simulink model "mcb_pmsm_foc_test_f28379d"  (R2023b)
settings: Solver=FixedStepDiscrete  StartTime=0.0  StopTime=10  RelTol=1e-3  EnableMultiTasking=on
InitFcn:
  | mcb_pmsm_foc_test_f28379d_data;
values from neighbouring files (symbols this model uses):
  dataType = 'single'    [mcb_pmsm_foc_sensorless_f28379d_datascript.m]    (also in mcb_pmsm_foc_test_f28379d_data.m)
  inverter = mcb_updateInverterParameters(pmsm,inverter,target)    [mcb_pmsm_foc_sensorless_f28379d_datascript.m]    (also in mcb_pmsm_foc_test_f28379d_data.m)
  PI_params = mcb_SetControllerParameters(pmsm,inverter,PU_System,T_pwm,2*Ts,Ts_speed)    [mcb_pmsm_foc_sensorless_f28379d_datascript.m]    (also in mcb_pmsm_foc_test_f28379d_data.m = mcb_SetControllerParameters(pmsm,inverter,PU_System,T_pwm,Ts)
  pmsm = mcb_SetPMSMMotorParameters("new")    [mcb_pmsm_foc_sensorless_f28379d_datascript.m]    (also in mcb_pmsm_foc_test_f28379d_data.m = mcb_SetPMSMMotorParameters("SF2804"))
  PU_System = mcb_SetPUSystem(pmsm,inverter)    [mcb_pmsm_foc_sensorless_f28379d_datascript.m]    (also in mcb_pmsm_foc_test_f28379d_data.m)
  target = mcb_SetProcessorDetails('F28379D',PWM_frequency)    [mcb_pmsm_foc_sensorless_f28379d_datascript.m]    (also in mcb_pmsm_foc_test_f28379d_data.m)
  Ts = T_pwm    [discrete_tansfer_fcn.m]    (also in mcb_pmsm_foc_sensorless_f28379d_datascript.m = 5e-05; mcb_pmsm_foc_test_f28379d_data.m = 5e-05)
  Ts_motor = T_pwm/2    (= 2.5e-05)    [mcb_pmsm_foc_sensorless_f28379d_datascript.m]    (also in mcb_pmsm_foc_test_f28379d_data.m)
  Ts_sensor = 20*Ts    (= 0.001)    [mcb_pmsm_foc_sensorless_f28379d_datascript.m]    (also in mcb_pmsm_foc_test_f28379d_data.m; virtual_speed.m)
  Ts_simulink = T_pwm/2    (= 2.5e-05)    [mcb_pmsm_foc_sensorless_f28379d_datascript.m]    (also in mcb_pmsm_foc_test_f28379d_data.m)
  Ts_speed = 20*Ts    (= 0.001)    [mcb_pmsm_foc_sensorless_f28379d_datascript.m]    (also in mcb_pmsm_foc_test_f28379d_data.m = 0.0005)
undefined symbols (not defined in the file or in its folder): DiscIntNeverNeededParam, Down, GPTRIP1SEL, GPTRIP2SEL, TZ1, TZ2, Up
libraries: c280xlib x14, simulink x11, mcbcontrolslib x9, c2802xlib x7, slpidlib x5, c2837xDlib x4, mcbpositiondecoderlib x3, canmsglib x2, svdschedulerlib x2, dspsigops x1, svdutilitieslib x1, mcbplantlib x1
(part 3 of 3)

== system mcb_pmsm_foc_test_f28379d/Serial Receive/SCI_Rx/Simulation ==
  Data Type Conversion2 : DataTypeConversion  OutDataTypeStr=dataType  RndMeth=Simplest  SaturateOnIntegerOverflow=off
  Data_Conditioning_Tx : Subsystem  Variant=on
  Debug_signals : Constant  OutDataTypeStr=uint16  SampleTime=-1
  Enable : Constant  OutDataTypeStr=uint16  SampleTime=-1
  Parse : Subsystem
  Reversal : Step  Time=3
  Speed_Ref_Final (rpm) : Constant  Value=-0.8*pmsm.N_base  OutDataTypeStr=dataType  SampleTime=-1
  Speed_Ref_Init (rpm) : Step  Before=0.2*pmsm.N_base  After=0.9*pmsm.N_base
  Switch : Switch  Criteria=u2 > Threshold  SaturateOnIntegerOverflow=off  InputSameDT=off
  rpm2PU : Gain  Gain=1/pmsm.N_base  RndMeth=Simplest  OutDataTypeStr=Inherit: Same as input
  Data : Outport
  wires:
  Data_Conditioning_Tx/1(Data) -> Data/1
  Parse/1(Data) -> Data_Conditioning_Tx/2(In2)
  Data Type Conversion2/1 -> Data_Conditioning_Tx/1(In1)
  Enable/1 -> Parse/1(Enable_PWM)
  Debug_signals/1 -> Parse/2(Debug_signals)
  rpm2PU/1 -> Data Type Conversion2/1
  Switch/1 -> rpm2PU/1
  Speed_Ref_Final (rpm)/1 -> Switch/1
  Reversal/1 -> Switch/2
  Speed_Ref_Init (rpm)/1 -> Switch/3

== system mcb_pmsm_foc_test_f28379d/Speed Control/PI_Controller_Speed1/Switch Case Action Subsystem ==
  Action Port : ActionPort  ActionPortLabel=case [ 1 ]:
  Constant : Constant  Value=0  OutDataTypeStr=single
  Constant1 : Constant  Value=0  OutDataTypeStr=single
  Constant2 : Constant  Value=0  OutDataTypeStr=boolean
  theta_virtual : Outport
  Iq_ref* : Outport  Port=2
  CloseLoop_Enable : Outport  Port=3
  wires:
  Constant/1 -> theta_virtual/1
  Constant1/1 -> Iq_ref*/1
  Constant2/1 -> CloseLoop_Enable/1

== system mcb_pmsm_foc_test_f28379d/Speed Control/PI_Controller_Speed1/Switch Case Action Subsystem1 ==
  Iq_ref : Inport
  Action Port : ActionPort  ActionPortLabel=case [ 2 ]:
  Constant : Constant  Value=0  OutDataTypeStr=single
  Constant2 : Constant  Value=0  OutDataTypeStr=boolean
  theta_virtual : Outport
  Iq_ref* : Outport  Port=2
  CloseLoop_Enable : Outport  Port=3
  wires:
  Constant/1 -> theta_virtual/1
  Iq_ref/1 -> Iq_ref*/1
  Constant2/1 -> CloseLoop_Enable/1

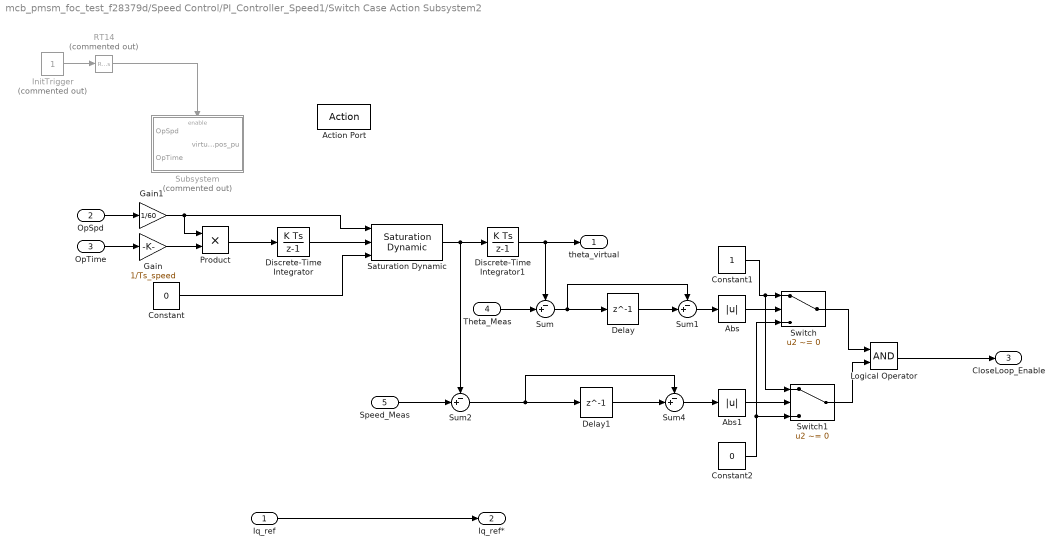
== system mcb_pmsm_foc_test_f28379d/Speed Control/PI_Controller_Speed1/Switch Case Action Subsystem2 ==
  Iq_ref : Inport
  OpSpd : Inport  Port=2
  OpTime : Inport  Port=3
  Theta_Meas : Inport  Port=4
  Speed_Meas : Inport  Port=5
  Action Port : ActionPort  ActionPortLabel=case [ 3 ]:
  Abs : Abs  SaturateOnIntegerOverflow=off
  Abs1 : Abs  SaturateOnIntegerOverflow=off
  Constant : Constant  Value=0
  Constant1 : Constant  OutDataTypeStr=boolean
  Constant2 : Constant  Value=0  OutDataTypeStr=boolean
  Delay : Delay  DelayLength=1  InitialCondition=0
  Delay1 : Delay  DelayLength=1  InitialCondition=0
  Discrete-Time Integrator : DiscreteIntegrator  SampleTime=-1  OutDataTypeStr=single  ICPrevOutput=DiscIntNeverNeededParam  ICPrevScaledInput=DiscIntNeverNeededParam
  Discrete-Time Integrator1 : DiscreteIntegrator  SampleTime=-1  OutDataTypeStr=single  ICPrevOutput=DiscIntNeverNeededParam  ICPrevScaledInput=DiscIntNeverNeededParam
  Gain : Gain  Gain=1/Ts_speed
  Gain1 : Gain  Gain=1/60
  InitTrigger : Constant  Priority=10  Commented=on  OutDataTypeStr=boolean
  Logical Operator : Logic  AllPortsSameDT=off  OutDataTypeStr=boolean
  Product : Product  OutDataTypeStr=single
  RT14 : RateTransition  Commented=on  Deterministic=off  OutPortSampleTime=Ts_sensor
  Saturation Dynamic : simulink/Discontinuities/Saturation Dynamic  OutMin=[]  OutMax=[]  OutDataTypeStr=single  OutDataType=fixdt(1, 16)  OutScaling=2^-10  DoSatur=off
  Subsystem : Subsystem  Commented=on
  Sum{,1..2,4} (4 alike) : Sum  Inputs=-+|
  Switch : Switch  Criteria=u2 ~= 0  SaturateOnIntegerOverflow=off  InputSameDT=off
  Switch1 : Switch  Criteria=u2 ~= 0  SaturateOnIntegerOverflow=off  InputSameDT=off
  theta_virtual : Outport
  Iq_ref* : Outport  Port=2
  CloseLoop_Enable : Outport  Port=3
  wires:
  Iq_ref/1 -> Iq_ref*/1
  InitTrigger/1 -> RT14/1
  RT14/1 -> Subsystem/Enable
  Constant/1 -> Saturation Dynamic/3
  OpSpd/1 -> Gain1/1
  Gain/1 -> Product/2
  OpTime/1 -> Gain/1
  Product/1 -> Discrete-Time Integrator/1
  Gain1/1 -> Saturation Dynamic/1, Product/1
  Discrete-Time Integrator/1 -> Saturation Dynamic/2
  Saturation Dynamic/1 -> Sum2/1, Discrete-Time Integrator1/1
  Discrete-Time Integrator1/1 -> Sum/1, theta_virtual/1
  Theta_Meas/1 -> Sum/2
  Speed_Meas/1 -> Sum2/2
  Sum/1 -> Sum1/1, Delay/1
  Delay/1 -> Sum1/2
  Sum1/1 -> Abs/1
  Abs/1 -> Switch/2
  Switch/1 -> Logical Operator/1
  Logical Operator/1 -> CloseLoop_Enable/1
  Switch1/1 -> Logical Operator/2
  Constant1/1 -> Switch1/1, Switch/1
  Abs1/1 -> Switch1/2
  Delay1/1 -> Sum4/2
  Constant2/1 -> Switch/3, Switch1/3
  Sum4/1 -> Abs1/1
  Sum2/1 -> Sum4/1, Delay1/1

== system mcb_pmsm_foc_test_f28379d/Speed Control/PI_Controller_Speed1/Switch Case Action Subsystem3 ==
  Iq_ref : Inport
  Action Port : ActionPort  ActionPortLabel=case [ 4 ]:
  Constant2 : Constant  Value=0  OutDataTypeStr=boolean
  theta_virtual : Outport
  Iq_ref* : Outport  Port=2
  CloseLoop_Enable : Outport  Port=3
  wires:
  ? -> theta_virtual/1
  Iq_ref/1 -> Iq_ref*/1
  Constant2/1 -> CloseLoop_Enable/1

== system mcb_pmsm_foc_test_f28379d/Speed Control/POS_Loop/Subsystem ==
  In1 : Inport
  Action Port : ActionPort  ActionPortLabel=if(u1 > 0.5)
  Fcn : Fcn  Expr=u(1)-1
  Out1 : Outport
  wires:
  In1/1 -> Fcn/1
  Fcn/1 -> Out1/1

== system mcb_pmsm_foc_test_f28379d/Speed Control/POS_Loop/Subsystem1 ==
  In1 : Inport
  Action Port : ActionPort  ActionPortLabel=elseif(u1 < -0.5)
  Fcn1 : Fcn  Expr=u(1)+1
  Out1 : Outport
  wires:
  Fcn1/1 -> Out1/1
  In1/1 -> Fcn1/1

== system mcb_pmsm_foc_test_f28379d/Speed Control/POS_Loop/Subsystem2 ==
  In1 : Inport
  Action Port : ActionPort  ActionPortLabel=else
  Out1 : Outport
  wires:
  In1/1 -> Out1/1

== system mcb_pmsm_foc_test_f28379d/AS5600 Read/Initialization/Delay 1ms/System Outputs ==

== system mcb_pmsm_foc_test_f28379d/Current Control/Control_System/Current_Controllers/PI_Controller_Id ==
  I_ref : Inport
  I_fb : Inport  Port=2
  Data Store Read1 : DataStoreRead  DataStoreName=Enable  IndexOptions=Index vector (dialog)  Indices=1  OutputSizes=1
  Discrete PI Controller with anti-windup & reset : slpidlib/PID Controller  Controller=PI  Form=Parallel  TimeDomain=Discrete-time  UseExternalTs=off  SampleTime=-1  IntegratorMethod=Forward Euler  FilterMethod=Forward Euler  ControllerParametersSource=external  P=1  I=1  UseKiTs=on  D=0  N=100  UseFilter=on  TunerSelectOption=Transfer Function Based (PID Tuner App)  InitialConditionSource=external  InitialConditionForIntegrator=0  InitialConditionForFilter=0  DifferentiatorICPrevScaledInput=0  ExternalReset=level  TrackingMode=off  Kt=1  LimitOutput=on  SatLimitsSource=internal  UpperSaturationLimit=1  LowerSaturationLimit=-1  LinearizeAsGain=on  AntiWindupMode=clamping  Kb=1  LimitIntegrator=off  UpperIntegratorSaturationLimit=inf  LowerIntegratorSaturationLimit=-inf  RndMeth=Simplest  POutMin=[]  POutMax=[]  IOutMin=[]  IOutMax=[]  DOutMin=[]  DOutMax=[]  NOutMin=[]  NOutMax=[]  SumOutMin=[]  SumOutMax=[]  SaturationOutDataTypeStr=Inherit: Inherit via back propagation  SaturationOutMin=[]  SaturationOutMax=[]  PParamMin=[]  PParamMax=[]  IParamMin=[]  IParamMax=[]  DParamMin=[]  DParamMax=[]  NParamMin=[]  NParamMax=[]  KbParamMin=[]  KbParamMax=[]  KtParamMin=[]  KtParamMax=[]  KbOutMin=[]  KbOutMax=[]  KtOutMin=[]  KtOutMax=[]  IntegratorOutMin=[]  IntegratorOutMax=[]  FilterOutMin=[]  FilterOutMax=[]  SumI1OutMin=[]  SumI1OutMax=[]  SumI2OutMin=[]  SumI2OutMax=[]  SumI3OutMin=[]  SumI3OutMax=[]  SumI4OutMin=[]  SumI4OutMax=[]  SumDOutMin=[]  SumDOutMax=[]  DifferentiatorOutMin=[]  DifferentiatorOutMax=[]  FilterDiffOutCoefMin=[]  FilterDiffOutCoefMax=[]  ReciprocalOutMin=[]  ReciprocalOutMax=[]  SumDenOutMin=[]  SumDenOutMax=[]  SumNumOutMin=[]  SumNumOutMax=[]  DivideOutMin=[]  DivideOutMax=[]  UdiffTsProdOutMin=[]  UdiffTsProdOutMax=[]  NTsProdOutMin=[]  NTsProdOutMax=[]  UintegralTsProdOutMin=[]  UintegralTsProdOutMax=[]  UngainTsProdOutMin=[]  UngainTsProdOutMax=[]  ClampingZeroOutDataTypeStr=Inherit: Inherit via back propagation  ClampingZeroOutMin=[]  ClampingZeroOutMax=[]  FilterDenConstantOutDataTypeStr=Inherit: Inherit via back propagation  FilterDenConstantOutMin=[]  FilterDenConstantOutMax=[]  PCopyOutDataTypeStr=Inherit: Inherit via back propagation  PCopyOutMin=[]  PCopyOutMax=[]  NCopyOutDataTypeStr=Inherit: Inherit via back propagation  NCopyOutMin=[]  NCopyOutMax=[]  IntegratorContinuousStateAttributes=''  IntegratorStateMustResolveToSignalObject=off  IntegratorRTWStateStorageClass=Auto  FilterContinuousStateAttributes=''  FilterStateMustResolveToSignalObject=off  FilterRTWStateStorageClass=Auto  ParallelPVariant=ExternalParameters  IdealPVariant=Disabled  IVariant=ExternalParameters  DVariant=Disabled  IntegratorVariant=Discrete  SatVariant=Enabled  AWVariant=DiscClampingParallel  PCopyVariant=Disabled  TRVariant=Disabled  FdbkBlocksVariant=Forward  IdealPFdbkVariant=Disabled  SatFdbkVariant=Disabled  DerivativeFilterVariant=Disabled  NVariant=Disabled  NCopyVariant=Disabled_SignalSpec  FilterICVariant=Disabled  IntegratorICVariant=ExternalICs  ExternalResetVariant=ExternalReset  TRSumVariant=Passthrough  SumFdbkVariant=Disabled  SumVariant=Sum_PI  TsampFilterVariant=InternalTs  TsampNgainVariant=Passthrough  TsampIntegralVariant=Disabled_SignalSpec  ExternalSaturationOutDataTypeStr=Inherit: Same as second input
      settings: LibrarySourceBlock=mcbcontrolslib/PI Controller
  Ki : Constant  Value=PI_params.Ki_id*Ts  OutDataTypeStr=dataType  SampleTime=-1
  Ki1 : Constant  Value=0  OutDataTypeStr=dataType  SampleTime=-1
  Kp : Constant  Value=PI_params.Kp_id  OutDataTypeStr=dataType  SampleTime=-1
  Logical Operator : Logic  Operator=NOT  IconShape=distinctive  AllPortsSameDT=off  OutDataTypeStr=boolean
  Sum : Sum  Inputs=|+-  OutDataTypeStr=Inherit: Same as first input
  V_ref : Outport  VectorParamsAs1DForOutWhenUnconnected=off
  wires:
  I_ref/1 -> Sum/1
  I_fb/1 -> Sum/2
  Data Store Read1/1 -> Logical Operator/1
  Discrete PI Controller with anti-windup & reset/1 -> V_ref/1
  Sum/1 -> Discrete PI Controller with anti-windup & reset/1
  Kp/1 -> Discrete PI Controller with anti-windup & reset/2
  Ki/1 -> Discrete PI Controller with anti-windup & reset/3
  Logical Operator/1 -> Discrete PI Controller with anti-windup & reset/4
  Ki1/1 -> Discrete PI Controller with anti-windup & reset/5

== system mcb_pmsm_foc_test_f28379d/Current Control/Control_System/Current_Controllers/PI_Controller_Iq ==
  I_ref : Inport
  I_fb : Inport  Port=2
  Data Store Read1 : DataStoreRead  DataStoreName=Enable  IndexOptions=Index vector (dialog)  Indices=1  OutputSizes=1
  Discrete PI Controller with anti-windup & reset : slpidlib/PID Controller  Controller=PI  Form=Parallel  TimeDomain=Discrete-time  UseExternalTs=off  SampleTime=-1  IntegratorMethod=Forward Euler  FilterMethod=Forward Euler  ControllerParametersSource=external  P=1  I=1  UseKiTs=on  D=0  N=100  UseFilter=on  TunerSelectOption=Transfer Function Based (PID Tuner App)  InitialConditionSource=external  InitialConditionForIntegrator=0  InitialConditionForFilter=0  DifferentiatorICPrevScaledInput=0  ExternalReset=level  TrackingMode=off  Kt=1  LimitOutput=on  SatLimitsSource=internal  UpperSaturationLimit=1  LowerSaturationLimit=-1  LinearizeAsGain=on  AntiWindupMode=clamping  Kb=1  LimitIntegrator=off  UpperIntegratorSaturationLimit=inf  LowerIntegratorSaturationLimit=-inf  RndMeth=Simplest  POutMin=[]  POutMax=[]  IOutMin=[]  IOutMax=[]  DOutMin=[]  DOutMax=[]  NOutMin=[]  NOutMax=[]  SumOutMin=[]  SumOutMax=[]  SaturationOutDataTypeStr=Inherit: Inherit via back propagation  SaturationOutMin=[]  SaturationOutMax=[]  PParamMin=[]  PParamMax=[]  IParamMin=[]  IParamMax=[]  DParamMin=[]  DParamMax=[]  NParamMin=[]  NParamMax=[]  KbParamMin=[]  KbParamMax=[]  KtParamMin=[]  KtParamMax=[]  KbOutMin=[]  KbOutMax=[]  KtOutMin=[]  KtOutMax=[]  IntegratorOutMin=[]  IntegratorOutMax=[]  FilterOutMin=[]  FilterOutMax=[]  SumI1OutMin=[]  SumI1OutMax=[]  SumI2OutMin=[]  SumI2OutMax=[]  SumI3OutMin=[]  SumI3OutMax=[]  SumI4OutMin=[]  SumI4OutMax=[]  SumDOutMin=[]  SumDOutMax=[]  DifferentiatorOutMin=[]  DifferentiatorOutMax=[]  FilterDiffOutCoefMin=[]  FilterDiffOutCoefMax=[]  ReciprocalOutMin=[]  ReciprocalOutMax=[]  SumDenOutMin=[]  SumDenOutMax=[]  SumNumOutMin=[]  SumNumOutMax=[]  DivideOutMin=[]  DivideOutMax=[]  UdiffTsProdOutMin=[]  UdiffTsProdOutMax=[]  NTsProdOutMin=[]  NTsProdOutMax=[]  UintegralTsProdOutMin=[]  UintegralTsProdOutMax=[]  UngainTsProdOutMin=[]  UngainTsProdOutMax=[]  ClampingZeroOutDataTypeStr=Inherit: Inherit via back propagation  ClampingZeroOutMin=[]  ClampingZeroOutMax=[]  FilterDenConstantOutDataTypeStr=Inherit: Inherit via back propagation  FilterDenConstantOutMin=[]  FilterDenConstantOutMax=[]  PCopyOutDataTypeStr=Inherit: Inherit via back propagation  PCopyOutMin=[]  PCopyOutMax=[]  NCopyOutDataTypeStr=Inherit: Inherit via back propagation  NCopyOutMin=[]  NCopyOutMax=[]  IntegratorContinuousStateAttributes=''  IntegratorStateMustResolveToSignalObject=off  IntegratorRTWStateStorageClass=Auto  FilterContinuousStateAttributes=''  FilterStateMustResolveToSignalObject=off  FilterRTWStateStorageClass=Auto  ParallelPVariant=ExternalParameters  IdealPVariant=Disabled  IVariant=ExternalParameters  DVariant=Disabled  IntegratorVariant=Discrete  SatVariant=Enabled  AWVariant=DiscClampingParallel  PCopyVariant=Disabled  TRVariant=Disabled  FdbkBlocksVariant=Forward  IdealPFdbkVariant=Disabled  SatFdbkVariant=Disabled  DerivativeFilterVariant=Disabled  NVariant=Disabled  NCopyVariant=Disabled_SignalSpec  FilterICVariant=Disabled  IntegratorICVariant=ExternalICs  ExternalResetVariant=ExternalReset  TRSumVariant=Passthrough  SumFdbkVariant=Disabled  SumVariant=Sum_PI  TsampFilterVariant=InternalTs  TsampNgainVariant=Passthrough  TsampIntegralVariant=Disabled_SignalSpec  ExternalSaturationOutDataTypeStr=Inherit: Same as second input
      settings: LibrarySourceBlock=mcbcontrolslib/PI Controller
  Ki : Constant  Value=PI_params.Ki_i*Ts  OutDataTypeStr=dataType  SampleTime=-1
  Kp : Constant  Value=PI_params.Kp_i  OutDataTypeStr=dataType  SampleTime=-1
  Kp1 : Constant  Value=0  OutDataTypeStr=dataType  SampleTime=-1
  Logical Operator : Logic  Operator=NOT  IconShape=distinctive  AllPortsSameDT=off  OutDataTypeStr=boolean
  Sum : Sum  Inputs=|+-  OutDataTypeStr=Inherit: Same as first input
  V_ref : Outport  VectorParamsAs1DForOutWhenUnconnected=off
  wires:
  Discrete PI Controller with anti-windup & reset/1 -> V_ref/1
  Data Store Read1/1 -> Logical Operator/1
  I_fb/1 -> Sum/2
  I_ref/1 -> Sum/1
  Kp/1 -> Discrete PI Controller with anti-windup & reset/2
  Sum/1 -> Discrete PI Controller with anti-windup & reset/1
  Ki/1 -> Discrete PI Controller with anti-windup & reset/3
  Logical Operator/1 -> Discrete PI Controller with anti-windup & reset/4
  Kp1/1 -> Discrete PI Controller with anti-windup & reset/5

== system mcb_pmsm_foc_test_f28379d/Current Control/Input Scaling/ Calculate Position and Speed/Subsystem ==
  In1 : Inport
  Action Port : ActionPort  ActionPortLabel=if(u1 > 0.5)
  Fcn : Fcn  Expr=u(1)-1
  Out1 : Outport
  wires:
  In1/1 -> Fcn/1
  Fcn/1 -> Out1/1

== system mcb_pmsm_foc_test_f28379d/Current Control/Input Scaling/ Calculate Position and Speed/Subsystem1 ==
  In1 : Inport
  Action Port : ActionPort  ActionPortLabel=elseif(u1 < -0.5)
  Fcn1 : Fcn  Expr=u(1)+1
  Out1 : Outport
  wires:
  Fcn1/1 -> Out1/1
  In1/1 -> Fcn1/1

== system mcb_pmsm_foc_test_f28379d/Current Control/Input Scaling/ Calculate Position and Speed/Subsystem2 ==
  In1 : Inport
  Action Port : ActionPort  ActionPortLabel=else
  Out1 : Outport
  wires:
  In1/1 -> Out1/1

== system mcb_pmsm_foc_test_f28379d/Current Control/Input Scaling/Calculate Phase Currents/Data_Type ==
  In1 : Inport
  Data_Type_Fixed_Point : Subsystem  VariantControl=~isequal(dataType,'single')
  Data_Type_Float : Subsystem  VariantControl=isequal(dataType,'single')
  Iab_meas_PU : Outport

== system mcb_pmsm_foc_test_f28379d/Current Control/SCI_Tx/Code Generation/Data_Conditioning_Tx ==
  In1 : Inport
  Data_Type_Fixed_Point : Subsystem  VariantControl=~isequal(dataType,'single')
  Data_Type_Float : Subsystem  VariantControl=isequal(dataType, 'single')
  Data_Log : Outport

== system mcb_pmsm_foc_test_f28379d/Current Control/SCI_Tx/Code Generation/Data_Logging ==
  note: Fast Serial Data Monitoring (32-bit)
  Data_Log : Inport
  Counter Limited : simulink/Sources/Counter Limited  uplimit=600-1  tsamp=-1
  Data : Subsystem  TreatAsAtomicUnit=on
  End : Subsystem  TreatAsAtomicUnit=on
  If : If  IfExpression=u1 == 0  ElseIfExpressions=u1 == 599
  Merge : Merge  Inputs=3
  Merge1 : Merge  Inputs=3
  Mux : Mux  Inputs=2
  Start : Subsystem  TreatAsAtomicUnit=on
  Width : Width  OutDataTypeMode=All ports same datatype  DataType=uint16
  SCI_Tx : Outport
  wires:
  If/3 -> Data/Action
  Data/1(Data_out) -> Merge/3
  Width/1 -> Data/2(Data_width), Start/2(Data_width), End/2(Data_width)
  Merge/1 -> Mux/1  "SCI_Tx_Data"
  Counter Limited/1 -> If/1
  Start/2(Iteration) -> Merge1/1
  Start/1(Data_out) -> Merge/1
  If/2 -> End/Action
  Merge1/1 -> Mux/2  "SCI_Tx_Iteration"
  If/1 -> Start/Action
  End/1(Data_out) -> Merge/2
  End/2(Iteration) -> Merge1/2
  Data/2(Iteration) -> Merge1/3
  Mux/1 -> SCI_Tx/1
  Data_Log/1 -> Width/1, Start/1(Data), End/1(Data), Data/1(Data)

== system mcb_pmsm_foc_test_f28379d/Current Control/SCI_Tx/Code Generation/While Iterator Subsystem ==
  Data : Inport
  Iteration : Inport  Port=2
  Add : Sum  Inputs=+-  OutDataTypeStr=Inherit: Same as first input
  Index Vector : MultiPortSwitch  Inputs=1  SaturateOnIntegerOverflow=off  InputSameDT=off
  SCI Transmit : c280xlib/SCI Transmit  sciModule=A  dataHead=''  dataTail=''  frameSize=1  blockingMode=on  outputStatus=off
  While Iterator : WhileIterator  MaxIters=-1  WhileBlockType=do-while  ShowIterationPort=on  OutputDataType=int16
  wires:
  While Iterator/1 -> Add/2, Index Vector/1
  Data/1 -> Index Vector/2
  Index Vector/1 -> SCI Transmit/1
  Add/1 -> While Iterator/1
  Iteration/1 -> Add/1

== system mcb_pmsm_foc_test_f28379d/Hardware Init/Variant Subsystem/Code Generation/Calculate ADC Offset  ==
  Enable : EnablePort
  Constant : Constant  Value=8
  Constant1 : Constant  Value=inverter.CtSensOffsetMax  OutDataTypeStr=Inherit: Inherit via back propagation
  Constant2 : Constant  Value=inverter.CtSensOffsetMin  OutDataTypeStr=Inherit: Inherit via back propagation
  Divide : Product  Inputs=*/  OutDataTypeStr=uint16
  Divide1 : Product  Inputs=*/  OutDataTypeStr=uint16
  For Iterator Subsystem : Subsystem  TreatAsAtomicUnit=on
  If : If  NumInputs=3  IfExpression=u1 > u3 & u1 < u2
  If Action Subsystem : Subsystem  TreatAsAtomicUnit=on
  If Action Subsystem1 : Subsystem  TreatAsAtomicUnit=on
  If Action Subsystem2 : Subsystem  TreatAsAtomicUnit=on
  If Action Subsystem3 : Subsystem  TreatAsAtomicUnit=on
  If1 : If  NumInputs=3  IfExpression=u1 > u3 & u1 < u2
  wires:
  If1/2 -> If Action Subsystem3/Action
  If1/1 -> If Action Subsystem2/Action
  Constant1/1 -> If1/2, If/2
  If/2 -> If Action Subsystem1/Action
  For Iterator Subsystem/1(Out1) -> Divide/1
  If/1 -> If Action Subsystem/Action
  Constant2/1 -> If1/3, If/3
  For Iterator Subsystem/2(Out2) -> Divide1/1
  Divide1/1 -> If1/1, If Action Subsystem2/1(In1)
  Constant/1 -> Divide1/2, Divide/2
  Divide/1 -> If Action Subsystem/1(In1), If/1

== system mcb_pmsm_foc_test_f28379d/Hardware Init/Variant Subsystem/Code Generation/DRV Enable ==
  note: Enable inverter
  In : Inport
  ADC Gain setting : Subsystem
  Constant : Constant  Value=inverter.EnableLogic
  Digital Output : c2837xDlib/Digital Output  Priority=10  GPIO_Number=GPIO120~GPIO127  GPIO_Bit0=off  GPIO_BIT0_Toggle=off  GPIO_Bit1=off  GPIO_BIT1_Toggle=off  GPIO_Bit2=off  GPIO_BIT2_Toggle=off  GPIO_Bit3=off  GPIO_BIT3_Toggle=off  GPIO_Bit4=on  GPIO_BIT4_Toggle=off  GPIO_Bit5=off  GPIO_BIT5_Toggle=off  GPIO_Bit6=off  GPIO_BIT6_Toggle=off  GPIO_Bit7=off  GPIO_BIT7_Toggle=off
  Digital Output1 : c2837xDlib/Digital Output  Priority=10  GPIO_Number=GPIO16~GPIO23  GPIO_Bit0=off  GPIO_BIT0_Toggle=off  GPIO_Bit1=off  GPIO_BIT1_Toggle=off  GPIO_Bit2=off  GPIO_BIT2_Toggle=off  GPIO_Bit3=off  GPIO_BIT3_Toggle=off  GPIO_Bit4=off  GPIO_BIT4_Toggle=off  GPIO_Bit5=off  GPIO_BIT5_Toggle=off  GPIO_Bit6=on  GPIO_BIT6_Toggle=off  GPIO_Bit7=off  GPIO_BIT7_Toggle=off
  Inverter Enable : Constant  OutDataTypeStr=uint16  SampleTime=-1
  NOT : Logic  Operator=NOT  IconShape=distinctive  AllPortsSameDT=off  OutDataTypeStr=boolean
  RunTimeMeasurement : Constant  OutDataTypeStr=uint16  SampleTime=-1
  Switch : Switch  Criteria=u2 > Threshold  SaturateOnIntegerOverflow=off  InputSameDT=off
  wires:
  Inverter Enable/1 -> Switch/1, NOT/1  "Active high logic for inverter enable"
  RunTimeMeasurement/1 -> Digital Output1/1
  Constant/1 -> ADC Gain setting/Enable, Switch/2
  Switch/1 -> Digital Output/1
  NOT/1 -> Switch/3  "Active low logic for inverter enable"
  In/1 -> ADC Gain setting/1(In1)

== system mcb_pmsm_foc_test_f28379d/Hardware Init/Variant Subsystem/Code Generation/Default ADC Offset ==
  Enable : EnablePort
  Constant : Constant  Value=inverter.CtSensAOffset  OutDataTypeStr=Inherit: Inherit via back propagation
  Constant1 : Constant  Value=inverter.CtSensBOffset  OutDataTypeStr=Inherit: Inherit via back propagation
  Data Store Write1 : DataStoreWrite  DataStoreName=IaOffset  IndexOptions=Index vector (dialog)  Indices=1  OutputSizes=1
  Data Store Write2 : DataStoreWrite  DataStoreName=IbOffset  IndexOptions=Index vector (dialog)  Indices=1  OutputSizes=1
  wires:
  Constant/1 -> Data Store Write1/1
  Constant1/1 -> Data Store Write2/1

== system mcb_pmsm_foc_test_f28379d/Serial Receive/SCI_Rx/Code Generation/Data_Type_Fixed_Point ==
  SCI Receive : c280xlib/SCI Receive  sciModule=A  dataHead=''  headerCheckMaxCount=16  dataTail=''  dataType=uint32  dataLenOptions=Length via dialog  dataDim=2  maxDataLength=1  initValue=0  errOption=Output the last received value  errValue=0  sampleTime=-1  blockingMode=on  timeOut=0.00875  outputStatus=off
  Data : Outport
  wires:
  SCI Receive/1 -> Data/1

== system mcb_pmsm_foc_test_f28379d/Serial Receive/SCI_Rx/Code Generation/Data_Type_Float ==
  SCI Receive : c280xlib/SCI Receive  sciModule=A  dataHead=''  headerCheckMaxCount=16  dataTail=''  dataType=single  dataLenOptions=Length via dialog  dataDim=2  maxDataLength=1  initValue=0  errOption=Output the last received value  errValue=0  sampleTime=-1  blockingMode=on  timeOut=0.00875  outputStatus=off
  Data : Outport
  wires:
  SCI Receive/1 -> Data/1

== system mcb_pmsm_foc_test_f28379d/Serial Receive/SCI_Rx/Simulation/Data_Conditioning_Tx ==
  In1 : Inport
  In2 : Inport  Port=2
  Data_Type_Fixed_Point : Subsystem  VariantControl=~isequal(dataType, 'single')
  Data_Type_Float : Subsystem  VariantControl=isequal(dataType, 'single')
  Data : Outport

== system mcb_pmsm_foc_test_f28379d/Serial Receive/SCI_Rx/Simulation/Parse ==
  Enable_PWM : Inport
  Debug_signals : Inport  Port=2
  Bitwise Operator : simulink/Logic and Bit Operations/Bitwise Operator  logicop=AND  UseBitMask=on  BitMask=hex2dec('0001')  BitMaskRealWorld=Stored Integer
  Bitwise Operator1 : simulink/Logic and Bit Operations/Bitwise Operator  logicop=AND  UseBitMask=on  BitMask=hex2dec('00F0')  BitMaskRealWorld=Stored Integer
  Shift Arithmetic1 : ArithShift  BitShiftNumber=-4
  Sum : Sum
  Data : Outport
  wires:
  Bitwise Operator/1 -> Sum/1
  Debug_signals/1 -> Shift Arithmetic1/1
  Sum/1 -> Data/1
  Shift Arithmetic1/1 -> Bitwise Operator1/1
  Enable_PWM/1 -> Bitwise Operator/1
  Bitwise Operator1/1 -> Sum/2

== system mcb_pmsm_foc_test_f28379d/Speed Control/PI_Controller_Speed1/Switch Case Action Subsystem2/Subsystem ==
  OpSpd : Inport
  OpTime : Inport  Port=2
  Enable : EnablePort
  Constant : Constant  Value=0
  Gain : Gain  Gain=1/Ts_speed
  MATLAB Function : MATLAB Function  TreatAsAtomicUnit=on
  Product : Product
  Saturation Dynamic : simulink/Discontinuities/Saturation Dynamic  OutMin=[]  OutMax=[]  OutDataTypeStr=Inherit: Same as second input  OutDataType=fixdt(1, 16)  OutScaling=2^-10  DoSatur=off
  Ts_sensor : Constant  Value=Ts_sensor
  virtual_pos_pu : Outport
  wires:
  MATLAB Function/1(pu) -> virtual_pos_pu/1
  Ts_sensor/1 -> MATLAB Function/2(Ts)
  Constant/1 -> Saturation Dynamic/3
  Product/1 -> Saturation Dynamic/2
  OpSpd/1 -> Saturation Dynamic/1, Product/1
  Saturation Dynamic/1 -> MATLAB Function/1(speed_ref_rpm)
  Gain/1 -> Product/2
  OpTime/1 -> Gain/1

== system mcb_pmsm_foc_test_f28379d/Current Control/Input Scaling/Calculate Phase Currents/Data_Type/Data_Type_Fixed_Point ==
  In1 : Inport
  Data Type Conversion : DataTypeConversion  OutDataTypeStr=fixdt(1,32,17)  ConvertRealWorld=Stored Integer (SI)  RndMeth=Simplest  SaturateOnIntegerOverflow=off
  Data Type Conversion1 : DataTypeConversion  OutDataTypeStr=dataType  RndMeth=Simplest  SaturateOnIntegerOverflow=off
  Q17 per unit conversion : ArithShift  BitShiftNumber=-6
  Iab_meas_PU : Outport
  wires:
  In1/1 -> Q17 per unit conversion/1
  Data Type Conversion1/1 -> Iab_meas_PU/1
  Data Type Conversion/1 -> Data Type Conversion1/1
  Q17 per unit conversion/1 -> Data Type Conversion/1

== system mcb_pmsm_foc_test_f28379d/Current Control/Input Scaling/Calculate Phase Currents/Data_Type/Data_Type_Float ==
  In1 : Inport
  Get ADC Voltage : Gain  Gain=target.ADC_Vref /target.ADC_MaxCount  OutDataTypeStr=dataType  RndMeth=Simplest
  Get Currents : Gain  Gain=1/inverter.ISenseVoltPerAmp  RndMeth=Simplest  OutDataTypeStr=Inherit: Same as input
  PU_Conversion : Gain  Gain=1/PU_System.I_base  RndMeth=Simplest  OutDataTypeStr=Inherit: Same as input
  Iab_meas_PU : Outport
  wires:
  PU_Conversion/1 -> Iab_meas_PU/1
  Get Currents/1 -> PU_Conversion/1
  Get ADC Voltage/1 -> Get Currents/1
  In1/1 -> Get ADC Voltage/1

== system mcb_pmsm_foc_test_f28379d/Current Control/SCI_Tx/Code Generation/Data_Conditioning_Tx/Data_Type_Fixed_Point ==
  In1 : Inport
  Data Type Conversion : DataTypeConversion  OutDataTypeStr=fixdt(1,32,28)  RndMeth=Simplest  SaturateOnIntegerOverflow=off
  Data Type Conversion3 : DataTypeConversion  OutDataTypeStr=uint32  ConvertRealWorld=Stored Integer (SI)  RndMeth=Simplest  SaturateOnIntegerOverflow=off
  Data_Log : Outport
  wires:
  In1/1 -> Data Type Conversion/1
  Data Type Conversion3/1 -> Data_Log/1
  Data Type Conversion/1 -> Data Type Conversion3/1

== system mcb_pmsm_foc_test_f28379d/Current Control/SCI_Tx/Code Generation/Data_Conditioning_Tx/Data_Type_Float ==
  In1 : Inport
  Byte Pack : svdutilitieslib/Byte Pack  maskPackedDataType=uint32  datatypes={'single'}  byteAlign=4  blockPlatform=tic2000
  Data_Log : Outport
  wires:
  Byte Pack/1 -> Data_Log/1
  In1/1 -> Byte Pack/1

== system mcb_pmsm_foc_test_f28379d/Current Control/SCI_Tx/Code Generation/Data_Logging/Data ==
  Data : Inport
  Data_width : Inport  Port=2
  Action Port : ActionPort  ActionPortLabel=else
  Dummy : Constant  Value=hex2dec('0000')  OutDataTypeStr=uint32
  Mux : Mux  Inputs=2
  Data_out : Outport  VectorParamsAs1DForOutWhenUnconnected=off
  Iteration : Outport  Port=2  VectorParamsAs1DForOutWhenUnconnected=off
  wires:
  Data_width/1 -> Iteration/1
  Data/1 -> Mux/1
  Dummy/1 -> Mux/2
  Mux/1 -> Data_out/1

== system mcb_pmsm_foc_test_f28379d/Current Control/SCI_Tx/Code Generation/Data_Logging/End ==
  Data : Inport
  Data_width : Inport  Port=2
  Action Port : ActionPort  ActionPortLabel=elseif(u1 == 599)
  Bias : Bias  Bias=1  SaturateOnIntegerOverflow=off
  End : Constant  Value=hex2dec('45454545')  OutDataTypeStr=uint32
  Mux : Mux  Inputs=2
  Data_out : Outport  VectorParamsAs1DForOutWhenUnconnected=off
  Iteration : Outport  Port=2  VectorParamsAs1DForOutWhenUnconnected=off
  wires:
  Data/1 -> Mux/1
  Data_width/1 -> Bias/1
  Bias/1 -> Iteration/1
  End/1 -> Mux/2
  Mux/1 -> Data_out/1

== system mcb_pmsm_foc_test_f28379d/Current Control/SCI_Tx/Code Generation/Data_Logging/Start ==
  Data : Inport
  Data_width : Inport  Port=2
  Action Port : ActionPort  ActionPortLabel=if(u1 == 0)
  Bias : Bias  Bias=1  SaturateOnIntegerOverflow=off
  Mux : Mux  Inputs=2
  Start : Constant  Value=hex2dec('53535353')  OutDataTypeStr=uint32
  Data_out : Outport  VectorParamsAs1DForOutWhenUnconnected=off
  Iteration : Outport  Port=2  VectorParamsAs1DForOutWhenUnconnected=off
  wires:
  Data/1 -> Mux/2
  Data_width/1 -> Bias/1
  Bias/1 -> Iteration/1
  Start/1 -> Mux/1
  Mux/1 -> Data_out/1

== system mcb_pmsm_foc_test_f28379d/Hardware Init/Variant Subsystem/Code Generation/Calculate ADC Offset /For Iterator Subsystem ==
  ADC_A_IN0 : c2802xlib/ADC  Priority=20  blkParamProc=C2000_Type4  ADCModule=C  samplingMode=Single sample mode  ADCResolution=12-bit (Single-ended input)  useSOC1=SOC2  useSOC2=SOC0_SOC1  SOCAcquisitionWindow=15  SOCTriggerSource=Software  SOCInterruptTrigger=No ADCINT  Ts=-1  dType=uint16  postInterrupt=off  interruptSel=ADCINT1  ADCINTContinuous=on  endma=off  chdma=1  conv1=ADCINA0  conv2=ADCINA0 and ADCINB0  conv1_Type4=ADCIN2  conv2_Type4=ADCIN0 and ADCIN1
  ADC_B_IN0 : c2802xlib/ADC  Priority=20  blkParamProc=C2000_Type4  ADCModule=B  samplingMode=Single sample mode  ADCResolution=12-bit (Single-ended input)  useSOC1=SOC2  useSOC2=SOC0_SOC1  SOCAcquisitionWindow=15  SOCTriggerSource=Software  SOCInterruptTrigger=No ADCINT  Ts=-1  dType=uint16  postInterrupt=off  interruptSel=ADCINT1  ADCINTContinuous=on  endma=off  chdma=1  conv1=ADCINA0  conv2=ADCINA0 and ADCINB0  conv1_Type4=ADCIN2  conv2_Type4=ADCIN0 and ADCIN1
  For Iterator : ForIterator  IterationLimit=16  IterationVariableDataType=uint16
  If : If  IfExpression=u1 > 8  ShowElse=off
  If Action Subsystem : Subsystem  TreatAsAtomicUnit=on
  Out1 : Outport
  Out2 : Outport  Port=2
  wires:
  For Iterator/1 -> If/1
  ADC_A_IN0/1 -> If Action Subsystem/1(In1)
  ADC_B_IN0/1 -> If Action Subsystem/2(In2)
  If Action Subsystem/1(Out1) -> Out1/1
  If Action Subsystem/2(Out2) -> Out2/1
  If/1 -> If Action Subsystem/Action

== system mcb_pmsm_foc_test_f28379d/Hardware Init/Variant Subsystem/Code Generation/Calculate ADC Offset /If Action Subsystem ==
  In1 : Inport
  Action Port : ActionPort  ActionPortLabel=if(u1 > u3 & u1 < u2)
  Data Store Write1 : DataStoreWrite  DataStoreName=IaOffset  IndexOptions=Index vector (dialog)  Indices=1  OutputSizes=1
  wires:
  In1/1 -> Data Store Write1/1

== system mcb_pmsm_foc_test_f28379d/Hardware Init/Variant Subsystem/Code Generation/Calculate ADC Offset /If Action Subsystem1 ==
  Action Port : ActionPort  ActionPortLabel=else
  Constant : Constant  Value=inverter.CtSensAOffset  OutDataTypeStr=Inherit: Inherit via back propagation
  Data Store Write1 : DataStoreWrite  DataStoreName=IaOffset  IndexOptions=Index vector (dialog)  Indices=1  OutputSizes=1
  wires:
  Constant/1 -> Data Store Write1/1

== system mcb_pmsm_foc_test_f28379d/Hardware Init/Variant Subsystem/Code Generation/Calculate ADC Offset /If Action Subsystem2 ==
  In1 : Inport
  Action Port : ActionPort  ActionPortLabel=if(u1 > u3 & u1 < u2)
  Data Store Write2 : DataStoreWrite  DataStoreName=IbOffset  IndexOptions=Index vector (dialog)  Indices=1  OutputSizes=1
  wires:
  In1/1 -> Data Store Write2/1

== system mcb_pmsm_foc_test_f28379d/Hardware Init/Variant Subsystem/Code Generation/Calculate ADC Offset /If Action Subsystem3 ==
  Action Port : ActionPort  ActionPortLabel=else
  Constant1 : Constant  Value=inverter.CtSensBOffset  OutDataTypeStr=Inherit: Inherit via back propagation
  Data Store Write2 : DataStoreWrite  DataStoreName=IbOffset  IndexOptions=Index vector (dialog)  Indices=1  OutputSizes=1
  wires:
  Constant1/1 -> Data Store Write2/1

== system mcb_pmsm_foc_test_f28379d/Hardware Init/Variant Subsystem/Code Generation/DRV Enable/ADC Gain setting ==
  In1 : Inport
  Enable : EnablePort
  Demux : Demux  Outputs=2
  Display : Display
      settings: Format=hex (Stored Integer)
  Display1 : Display
      settings: Format=hex (Stored Integer)
  SPI Master Transfer : c280xlib/SPI Controller Transfer  SPISelect=SPI_A  ClockPolarity=Rising_edge  ClockPhase=No_delay  SPIModule=uint32(0)  Mode=Master  BusSpeed=uint32(1000000)  FirstBitToTransfer=Most significant bit (MSB)  ClockMode=0  BlockFunction=Transfer  EnableRegisterAddress=off  RegisterAddress=0  OutputDataType=int8  OutputDataLength=1  DataBits=16  UseCustomSSPin=Provided by the SPI peripheral  ActiveLowSSPin=Active low  Pin=61
  SPI Master Transfer1 : c280xlib/SPI Controller Transfer  SPISelect=SPI_A  ClockPolarity=Rising_edge  ClockPhase=No_delay  SPIModule=uint32(0)  Mode=Master  BusSpeed=uint32(1000000)  FirstBitToTransfer=Most significant bit (MSB)  ClockMode=0  BlockFunction=Transfer  EnableRegisterAddress=off  RegisterAddress=0  OutputDataType=int8  OutputDataLength=1  DataBits=16  UseCustomSSPin=Provided by the SPI peripheral  ActiveLowSSPin=Active low  Pin=61
  wires:
  SPI Master Transfer1/1 -> Display1/1
  Demux/2 -> SPI Master Transfer1/1
  In1/1 -> Demux/1
  SPI Master Transfer/1 -> Display/1
  Demux/1 -> SPI Master Transfer/1

== system mcb_pmsm_foc_test_f28379d/Serial Receive/SCI_Rx/Simulation/Data_Conditioning_Tx/Data_Type_Fixed_Point ==
  In1 : Inport
  In2 : Inport  Port=2
  Data Type Conversion : DataTypeConversion  OutDataTypeStr=fixdt(1,32,28)  RndMeth=Simplest  SaturateOnIntegerOverflow=off
  Data Type Conversion1 : DataTypeConversion  OutDataTypeStr=uint32  RndMeth=Simplest  SaturateOnIntegerOverflow=off
  Data Type Conversion3 : DataTypeConversion  OutDataTypeStr=uint32  ConvertRealWorld=Stored Integer (SI)  RndMeth=Simplest  SaturateOnIntegerOverflow=off
  Mux : Mux  Inputs=2
  Data : Outport
  wires:
  In1/1 -> Data Type Conversion/1
  Data Type Conversion3/1 -> Mux/1
  Data Type Conversion/1 -> Data Type Conversion3/1
  In2/1 -> Data Type Conversion1/1
  Data Type Conversion1/1 -> Mux/2
  Mux/1 -> Data/1

== system mcb_pmsm_foc_test_f28379d/Serial Receive/SCI_Rx/Simulation/Data_Conditioning_Tx/Data_Type_Float ==
  In1 : Inport
  In2 : Inport  Port=2
  Data Type Conversion2 : DataTypeConversion  OutDataTypeStr=single  RndMeth=Simplest  SaturateOnIntegerOverflow=off
  Mux : Mux  Inputs=2
  Data : Outport
  wires:
  In1/1 -> Mux/1
  Mux/1 -> Data/1
  In2/1 -> Data Type Conversion2/1
  Data Type Conversion2/1 -> Mux/2

== system mcb_pmsm_foc_test_f28379d/Hardware Init/Variant Subsystem/Code Generation/Calculate ADC Offset /For Iterator Subsystem/If Action Subsystem ==
  In1 : Inport
  In2 : Inport  Port=2
  Action Port : ActionPort  ActionPortLabel=if(u1 > 8)
  Memory : Memory  InheritSampleTime=on
  Memory1 : Memory  InheritSampleTime=on
  Sum : Sum
  Sum1 : Sum
  Out1 : Outport
  Out2 : Outport  Port=2
  wires:
  In1/1 -> Sum/1
  Sum/1 -> Out1/1, Memory/1
  In2/1 -> Sum1/1
  Memory/1 -> Sum/2
  Sum1/1 -> Out2/1, Memory1/1
  Memory1/1 -> Sum1/2

== matlab function mcb_pmsm_foc_test_f28379d/AS5600 Read/Data Realignment /MATLAB Function ==
  data: data input; raw_angle output
function raw_angle = fcn(data)
    %#codegen
    
    % 提取 MSB 和 LSB
    msb = data(1);
    lsb = data(2);
    
    % 合并 MSB 和 LSB 到一个 16-bit 整数
    raw_angle = bitshift(uint16(msb), 8) + uint16(lsb);
    
end

== matlab function mcb_pmsm_foc_test_f28379d/Subsystem/MATLAB Function ==
  data: speed_ref_rpm input; pu output; Ts input
function pu = periodic_pu_pos(speed_ref_rpm, Ts)
% 根据参考转速生成周期变化的转子位置标幺值
% 入口：
%   speed_ref_rpm - 参考转速（rpm）
%   Ts            - 调用周期（s）
% 出口：
%   pu            - 转子位置 0~1

persistent theta
if isempty(theta), theta = 0; end

% 每拍走过的“转数”
delta = (speed_ref_rpm/60)*Ts;   % rpm -> rps -> 转/拍

theta = mod(theta + delta, 1);   % 积分并归一化
pu    = single(theta);
end

== stateflow chart mcb_pmsm_foc_test_f28379d/Speed Control/PI_Controller_Speed1/Chart ==
  state IDLE
    Motor_State = 1;
  state AlignStage
    Motor_State = 2;
  state OpenStage
    Motor_State = 3;
  state RunStage
    Motor_State = 4;
  note: &&CloseLoop_Enable==true
  (default) -> IDLE
  IDLE -> AlignStage : [Motor_Enable==true]
  AlignStage -> OpenStage [order 2] : [after(1000,tick)]
  OpenStage -> RunStage [order 1] : [after(4000,tick)]
  OpenStage -> IDLE [order 2] : [Motor_Enable==false]
  RunStage -> IDLE : [Motor_Enable==false]
  AlignStage -> IDLE [order 1] : [Motor_Enable==false]
  data: Motor_State output; Motor_Enable input; CloseLoop_Enable input

== matlab function mcb_pmsm_foc_test_f28379d/Speed Control/PI_Controller_Speed1/Switch Case Action Subsystem2/Subsystem/MATLAB Function ==
  data: speed_ref_rpm input; pu output; Ts input
function pu = periodic_pu_pos(speed_ref_rpm, Ts)
% 根据参考转速生成周期变化的转子位置标幺值
% 入口：
%   speed_ref_rpm - 参考转速（rpm）
%   Ts            - 调用周期（s）
% 出口：
%   pu            - 转子位置 0~1

persistent theta
if isempty(theta), theta = 0; end

% 每拍走过的“转数”
delta = (speed_ref_rpm/60)*Ts;   % rpm -> rps -> 转/拍

theta = mod(theta + delta, 1);   % 积分并归一化
pu    = single(theta);
end
